simulink model "PMSMDriveThermal"  (R2025b)
settings: Solver=ode15s  StartTime=0.0  StopTime=1  MaxStep=1e-3  MinStep=1e-10  RelTol=1e-2  AbsTol=1e-6  EnableMultiTasking=on
PreLoadFcn:
  | PMSMDriveThermalData;
values from neighbouring files (symbols this model uses):
  N = 6    [E25runs1.mat]
  PM = 0.03    [E25runs1.mat]
undefined symbols (not defined in the file or in its folder): f_losses, Isc_losses, losses_oc, losses_sc
libraries: batteryecm_lib x280, fl_lib x53, nesl_utility x21, ee_lib x10, SimscapeFluids_lib x3, eePmsmFieldOrientedControl x1
(part 24 of 24)

== system PMSMDriveThermal/Cooling system /Sensing Temperature Inverter ==
  PS-Simulink Converter : nesl_utility/PS-Simulink Converter  PhysicalDomain=network_engine_domain  SubClassName=ps_output  LeftPortType=input  RightPortType=output  PseudoPeriodic=off  Frequencies=[]  VectorFormat=1-D array  Unit=degC  AffineConversion=on
  Temperature Sensor : fl_lib/Thermal/Thermal Sensors/Temperature Sensor  temperature_measure=foundation.enum.MeasurementReference.difference
  ThRef : fl_lib/Thermal/Thermal Elements/Thermal Reference
  H : PMIOPort  Side=Left
  Cooling Inverter : Outport
  wires:
  PS-Simulink Converter/1 -> Cooling Inverter/1
  connections:
  ThRef/LConn1 -- Temperature Sensor/RConn1
  H/RConn1 -- Temperature Sensor/LConn1
  Temperature Sensor/RConn2 -- PS-Simulink Converter/LConn1

== system PMSMDriveThermal/Cooling system /Subsystem ==
  "Motor Temp " : Scope
      settings: ActiveDisplayYMinimum=24.999993193295392  ActiveDisplayYMaximum=25.000005404995338  DataLoggingVariableName=ScopeData2
  PS-Simulink Converter : nesl_utility/PS-Simulink Converter  PhysicalDomain=network_engine_domain  SubClassName=ps_output  LeftPortType=input  RightPortType=output  PseudoPeriodic=off  Frequencies=[]  VectorFormat=inherit  Unit=degC  AffineConversion=on
  Temperature Sensor : fl_lib/Thermal/Thermal Sensors/Temperature Sensor  temperature_measure=foundation.enum.MeasurementReference.difference
  Thermal Reference : fl_lib/Thermal/Thermal Elements/Thermal Reference
  Conn1 : PMIOPort  Side=Left
  wires:
  PS-Simulink Converter/1 -> "Motor Temp "/1  "Motor Temperature"
  connections:
  Temperature Sensor/LConn1 -- Conn1/RConn1
  Thermal Reference/LConn1 -- Temperature Sensor/RConn1
  PS-Simulink Converter/LConn1 -- Temperature Sensor/RConn2

== system PMSMDriveThermal/Scopes/losses ==
  idq : Inport
  w : Inport  Port=2
  Demux : Demux  Outputs=2
  MATLAB Function : MATLAB Function  TreatAsAtomicUnit=on
  tq_loss : Outport
  wires:
  w/1 -> MATLAB Function/3(w)
  MATLAB Function/1(trq_loss) -> tq_loss/1
  idq/1 -> Demux/1
  Demux/1 -> MATLAB Function/1(i_d)
  Demux/2 -> MATLAB Function/2(i_q)

== system PMSMDriveThermal/Thermal model/Sensing Temperature Rot ==
  PS-Simulink Converter : nesl_utility/PS-Simulink Converter  PhysicalDomain=network_engine_domain  SubClassName=ps_output  LeftPortType=input  RightPortType=output  PseudoPeriodic=off  Frequencies=[]  VectorFormat=1-D array  Unit=degC  AffineConversion=on
  Temperature Sensor : fl_lib/Thermal/Thermal Sensors/Temperature Sensor  temperature_measure=foundation.enum.MeasurementReference.difference
  ThRef : fl_lib/Thermal/Thermal Elements/Thermal Reference
  H : PMIOPort  Side=Left
  tag scope: TR=global
  wires:
  PS-Simulink Converter/1 -> [TR]
  connections:
  Temperature Sensor/RConn2 -- PS-Simulink Converter/LConn1
  ThRef/LConn1 -- Temperature Sensor/RConn1
  H/RConn1 -- Temperature Sensor/LConn1

== system PMSMDriveThermal/Thermal model/Sensing Temperature WiA ==
  PS-Simulink Converter : nesl_utility/PS-Simulink Converter  PhysicalDomain=network_engine_domain  SubClassName=ps_output  LeftPortType=input  RightPortType=output  PseudoPeriodic=off  Frequencies=[]  VectorFormat=1-D array  Unit=degC  AffineConversion=on
  Temperature Sensor : fl_lib/Thermal/Thermal Sensors/Temperature Sensor  temperature_measure=foundation.enum.MeasurementReference.difference
  ThRef : fl_lib/Thermal/Thermal Elements/Thermal Reference
  H : PMIOPort  Side=Left
  tag scope: TA=global
  wires:
  PS-Simulink Converter/1 -> [TA]
  connections:
  H/RConn1 -- Temperature Sensor/LConn1
  ThRef/LConn1 -- Temperature Sensor/RConn1
  Temperature Sensor/RConn2 -- PS-Simulink Converter/LConn1

== system PMSMDriveThermal/Thermal model/Sensing Temperature WiB ==
  PS-Simulink Converter : nesl_utility/PS-Simulink Converter  PhysicalDomain=network_engine_domain  SubClassName=ps_output  LeftPortType=input  RightPortType=output  PseudoPeriodic=off  Frequencies=[]  VectorFormat=1-D array  Unit=degC  AffineConversion=on
  Temperature Sensor : fl_lib/Thermal/Thermal Sensors/Temperature Sensor  temperature_measure=foundation.enum.MeasurementReference.difference
  ThRef : fl_lib/Thermal/Thermal Elements/Thermal Reference
  H : PMIOPort  Side=Left
  tag scope: TB=global
  wires:
  PS-Simulink Converter/1 -> [TB]
  connections:
  ThRef/LConn1 -- Temperature Sensor/RConn1
  H/RConn1 -- Temperature Sensor/LConn1
  Temperature Sensor/RConn2 -- PS-Simulink Converter/LConn1

== system PMSMDriveThermal/Thermal model/Sensing Temperature WiC ==
  PS-Simulink Converter : nesl_utility/PS-Simulink Converter  PhysicalDomain=network_engine_domain  SubClassName=ps_output  LeftPortType=input  RightPortType=output  PseudoPeriodic=off  Frequencies=[]  VectorFormat=1-D array  Unit=degC  AffineConversion=on
  Temperature Sensor : fl_lib/Thermal/Thermal Sensors/Temperature Sensor  temperature_measure=foundation.enum.MeasurementReference.difference
  ThRef : fl_lib/Thermal/Thermal Elements/Thermal Reference
  H : PMIOPort  Side=Left
  tag scope: TC=global
  wires:
  PS-Simulink Converter/1 -> [TC]
  connections:
  H/RConn1 -- Temperature Sensor/LConn1
  ThRef/LConn1 -- Temperature Sensor/RConn1
  Temperature Sensor/RConn2 -- PS-Simulink Converter/LConn1

== matlab function PMSMDriveThermal/Scopes/losses/MATLAB Function ==
  data: i_d input; trq_loss output; i_q input; w input; PM parameter; N parameter; losses_oc parameter; losses_sc parameter; f_losses parameter; Isc_losses parameter
function trq_loss = fcn(i_d,i_q,w,PM, N, losses_oc, losses_sc, f_losses, Isc_losses)

lambda = 2*pi*PM/(sqrt(2)*N);
a_h = losses_oc(1)/f_losses;
a_J = losses_oc(2)/f_losses^2;
a_ex = losses_oc(3)/f_losses^1.5;

b_h = losses_sc(1)/f_losses;
b_J = losses_sc(2)/f_losses^2;
b_ex = losses_sc(3)/f_losses^1.5;

Id = abs(i_d)/sqrt(2);
w_abs = abs(w);
if Id>0.999*Isc_losses
    ratio_Id_Isc = 0.999;
else
    ratio_Id_Isc = Id/Isc_losses;
end
Vd = lambda*w_abs*N/(2*pi)*ratio_Id_Isc; 
Iq = abs(i_q)/sqrt(2);
Vm = lambda*w_abs*N/(2*pi)*sqrt((1-ratio_Id_Isc)^2+(Iq/Isc_losses)^2);

Vm_losses = a_h/lambda*Vm+a_J/lambda^2*Vm^2+a_ex/lambda^1.5*Vm^1.5;
Vd_losses = b_h/lambda*Vd+b_J/lambda^2*Vd^2+b_ex/lambda^1.5*Vd^1.5;

trq_loss = sign(w)*(Vd_losses+Vm_losses)/(w_abs+1);
